simulink model "gm_sampleModel1871_2_sub"  (R2023a)
settings: Solver=VariableStepAuto  StartTime=0.0  StopTime=10.0  RelTol=1e-3
libraries: hdlsllib x1
settings Model: Creator=user1  LastModifiedBy=user1
settings OptimizationCC: BlockReduction=off  ConditionallyExecuteInputs=off
settings DebuggingCC: InheritedTsInSrcMsg=none

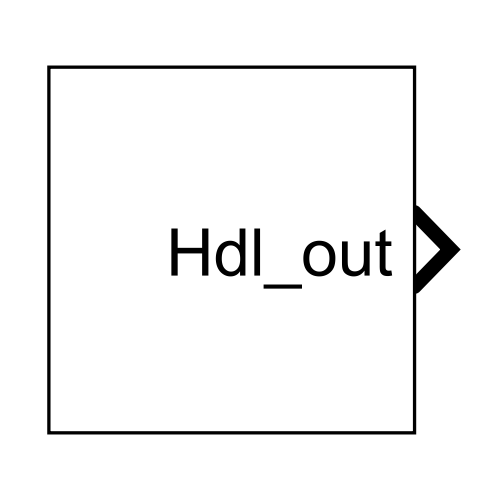
[thumbnail: Simulink's stored preview of the top-level diagram]
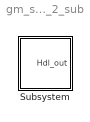
== system gm_sampleModel1871_2_sub ==
  Subsystem : Subsystem

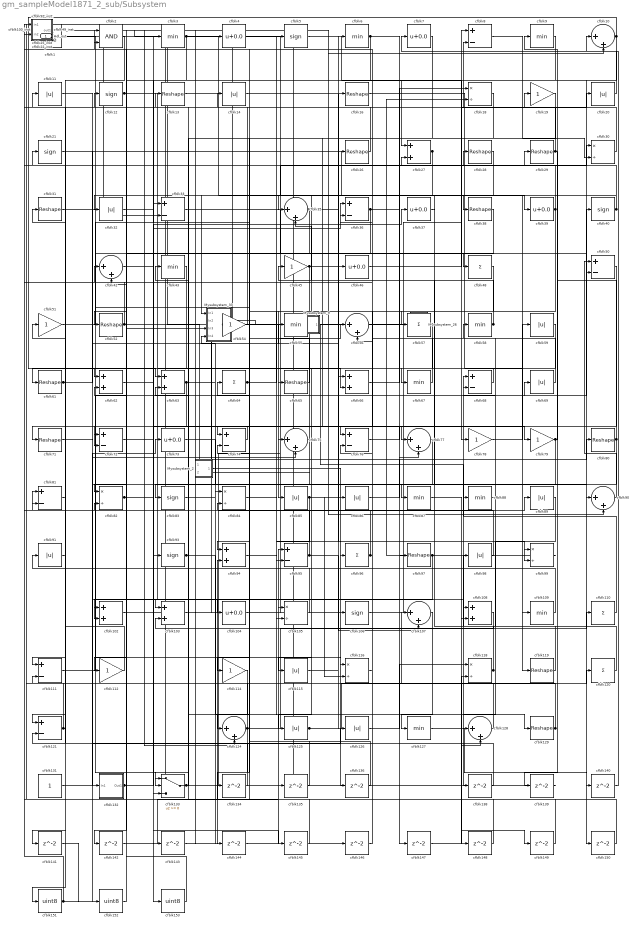
== system gm_sampleModel1871_2_sub/Subsystem ==
  Mysubsystem_2 : Subsystem
  Mysubsystem_26 : Subsystem
  Mysubsystem_33 : Subsystem
  Mysubsystem_9 : Subsystem
  cfblk1 : hdlsllib/Logic and Bit Operations/Bit Slice  lidx=7  ridx=0
  cfblk{10,35,42,56,75,77,90,107,124,128} (10 alike) : Sum  Inputs=|++  OutDataTypeStr=uint8
  cfblk100_inst : Subsystem
  cfblk{27,62..63,66,94,102..103,108} (8 alike) : Sum  OutDataTypeStr=uint8
  cfblk{4,7,37,39,46,73,104} (7 alike) : Bias  Bias=0.0  SaturateOnIntegerOverflow=off
  cfblk{18,30,82,84,99,105,116,118} (8 alike) : Product  Inputs=*/  OutDataTypeStr=uint8  RndMeth=Zero  SaturateOnIntegerOverflow=on
  cfblk{5,12,21,40,83,93,106} (7 alike) : Signum
  cfblk{3,6,9,43,55,58,67,87..88,109,127} (11 alike) : MinMax  OutDataTypeStr=uint8
  cfblk{11,14,20,32,59,69,85..86,89,91,98,115,125..126} (14 alike) : Abs  OutDataTypeStr=uint8  SaturateOnIntegerOverflow=off
  cfblk{48,57,64,96,110,120} (6 alike) : Sum  Inputs=+  OutDataTypeStr=uint8
  cfblk{8,33,36,50,68,72,74,76,81,95,111,121} (12 alike) : Sum  Inputs=+-  OutDataTypeStr=uint8
  cfblk{19,45,51,54,78..79,112,114} (8 alike) : Gain  OutDataTypeStr=uint8
  cfblk{13,16,26,28..29,31,38,52,61,65,71,80,97,119,129} (15 alike) : Reshape
  cfblk122_inst : Subsystem
  cfblk131 : Constant  OutDataTypeStr=uint8  SampleTime=-1
  cfblk132 : Subsystem
  cfblk133 : Switch  OutDataTypeStr=uint8  SaturateOnIntegerOverflow=off  InputSameDT=off
  cfblk{134..136,138..150} (16 alike) : Delay  SampleTime=1
  cfblk151 : DataTypeConversion  OutDataTypeStr=uint8  SaturateOnIntegerOverflow=off  RndMeth=Floor
  cfblk152 : DataTypeConversion  OutDataTypeStr=uint8  SaturateOnIntegerOverflow=off  RndMeth=Floor
  cfblk153 : DataTypeConversion  OutDataTypeStr=uint8  SaturateOnIntegerOverflow=off  RndMeth=Floor
  cfblk2 : Logic  AllPortsSameDT=off  OutDataTypeStr=boolean
  cfblk22_inst : Subsystem
  cfblk25_inst : Subsystem
  cfblk49_inst : Subsystem
  cfblk92_inst : Subsystem
  Hdl_out : Outport  OutDataTypeStr=uint8  SampleTime=1
  wires:
  Mysubsystem_2/1(Out2) -> cfblk136/1
  Mysubsystem_26/1(Out1) -> Mysubsystem_2/2(In2)
  Mysubsystem_33/1(Out1) -> Mysubsystem_2/1(In1)
  Mysubsystem_9/1(Out2) -> cfblk138/1
  cfblk1/1 -> cfblk74/1, cfblk133/2, cfblk116/1
  cfblk10/1 -> cfblk62/1, cfblk27/1, cfblk150/1
  cfblk100_inst/1(out1) -> cfblk90/2, cfblk106/1
  cfblk102/1 -> Mysubsystem_9/1(In2)
  cfblk103/1 -> cfblk56/1
  cfblk104/1 -> cfblk29/1
  cfblk105/1 -> cfblk91/1
  cfblk106/1 -> Mysubsystem_26/1(In1)
  cfblk107/1 -> cfblk127/1
  cfblk108/1 -> cfblk103/2
  cfblk109/1 -> cfblk64/1
  cfblk11/1 -> cfblk132/1(In1)
  cfblk110/1 -> cfblk68/1
  cfblk111/1 -> cfblk40/1
  cfblk112/1 -> cfblk31/1
  cfblk114/1 -> cfblk22_inst/1(in1)
  cfblk115/1 -> cfblk89/1
  cfblk116/1 -> cfblk36/1
  cfblk118/1 -> cfblk98/1, cfblk84/2
  cfblk119/1 -> cfblk45/1
  cfblk12/1 -> cfblk66/2, cfblk148/1
  cfblk120/1 -> cfblk68/2
  cfblk121/1 -> cfblk92_inst/2(in2), cfblk81/1
  cfblk122_inst/1(out1) -> cfblk33/2
  cfblk124/1 -> cfblk51/1, cfblk144/1, cfblk110/1
  cfblk125/1 -> cfblk86/1, cfblk120/1
  cfblk126/1 -> cfblk118/1
  cfblk127/1 -> cfblk140/1
  cfblk128/1 -> cfblk107/1
  cfblk129/1 -> cfblk11/1, Mysubsystem_33/4(In4)
  cfblk13/1 -> cfblk39/1
  cfblk131/1 -> cfblk73/1
  cfblk132/1(Out1) -> cfblk93/1, cfblk37/1
  cfblk133/1 -> cfblk63/2, cfblk16/1
  cfblk134/1 -> cfblk81/2
  cfblk135/1 -> cfblk111/2
  cfblk136/1 -> cfblk22_inst/2(in2)
  cfblk138/1 -> cfblk121/2
  cfblk139/1 -> cfblk1/1
  cfblk14/1 -> cfblk46/1
  cfblk140/1 -> cfblk10/1
  cfblk141/1 -> cfblk152/1
  cfblk142/1 -> cfblk95/1
  cfblk143/1 -> cfblk84/1
  cfblk144/1 -> cfblk105/1
  cfblk145/1 -> cfblk49_inst/1(in1)
  cfblk146/1 -> cfblk76/2
  cfblk147/1 -> cfblk118/2
  cfblk148/1 -> cfblk62/2
  cfblk149/1 -> cfblk94/2
  cfblk150/1 -> cfblk74/2
  cfblk151/1 -> cfblk75/2, cfblk126/1, cfblk100_inst/2(in2)
  cfblk152/1 -> cfblk2/1
  cfblk153/1 -> cfblk2/2
  cfblk16/1 -> cfblk119/1
  cfblk18/1 -> cfblk134/1
  cfblk19/1 -> cfblk103/1
  cfblk2/1 -> cfblk151/1
  cfblk20/1 -> cfblk7/1
  cfblk21/1 -> cfblk77/2
  cfblk22_inst/1(out1) -> cfblk135/1, Mysubsystem_33/3(In3)
  cfblk25_inst/1(out1) -> cfblk124/2
  cfblk26/1 -> cfblk122_inst/2(in2)
  cfblk27/1 -> cfblk85/1, Mysubsystem_33/1(In1)
  cfblk28/1 -> cfblk67/1
  cfblk29/1 -> cfblk8/2, cfblk139/1
  cfblk3/1 -> cfblk38/1, cfblk133/3
  cfblk30/1 -> cfblk14/1
  cfblk31/1 -> cfblk48/1
  cfblk32/1 -> cfblk77/1
  cfblk33/1 -> cfblk97/1
  cfblk35/1 -> cfblk102/2, cfblk30/1
  cfblk36/1 -> cfblk50/2, cfblk142/1
  cfblk37/1 -> cfblk87/1
  cfblk38/1 -> cfblk94/1
  cfblk39/1 -> cfblk95/2, cfblk35/1, cfblk27/2
  cfblk4/1 -> cfblk109/1
  cfblk40/1 -> cfblk49_inst/2(in2), cfblk32/1
  cfblk42/1 -> cfblk143/1
  cfblk43/1 -> cfblk112/1
  cfblk45/1 -> cfblk102/1, cfblk99/2
  cfblk46/1 -> cfblk20/1
  cfblk48/1 -> cfblk76/1
  cfblk49_inst/1(out1) -> cfblk4/1, cfblk25_inst/2(in2), cfblk10/2
  cfblk5/1 -> cfblk78/1
  cfblk50/1 -> cfblk141/1
  cfblk51/1 -> cfblk3/1
  cfblk52/1 -> cfblk92_inst/1(in1), cfblk82/1, cfblk147/1
  cfblk54/1 -> cfblk12/1
  cfblk55/1 -> cfblk100_inst/1(in1), cfblk18/2, Mysubsystem_33/2(In2)
  cfblk56/1 -> cfblk8/1
  cfblk57/1 -> cfblk121/1, Hdl_out/1
  cfblk58/1 -> cfblk35/2, cfblk57/1
  cfblk59/1 -> cfblk125/1
  cfblk6/1 -> cfblk72/2, cfblk108/1
  cfblk61/1 -> cfblk63/1, cfblk26/1, cfblk108/2, cfblk55/1
  cfblk62/1 -> cfblk153/1
  cfblk63/1 -> cfblk72/1, cfblk65/1
  cfblk64/1 -> cfblk5/1, cfblk99/1
  cfblk65/1 -> cfblk33/1
  cfblk66/1 -> cfblk18/1
  cfblk67/1 -> cfblk122_inst/1(in1)
  cfblk68/1 -> cfblk61/1
  cfblk69/1 -> cfblk42/1
  cfblk7/1 -> cfblk75/1
  cfblk71/1 -> cfblk88/1
  cfblk72/1 -> cfblk145/1
  cfblk73/1 -> cfblk90/1
  cfblk74/1 -> cfblk71/1
  cfblk75/1 -> cfblk114/1
  cfblk76/1 -> cfblk79/1
  cfblk77/1 -> cfblk124/1
  cfblk78/1 -> cfblk59/1
  cfblk79/1 -> cfblk133/1, cfblk9/1
  cfblk8/1 -> cfblk30/2
  cfblk80/1 -> cfblk83/1, cfblk19/1
  cfblk81/1 -> cfblk111/1
  cfblk82/1 -> cfblk42/2, cfblk36/2
  cfblk83/1 -> cfblk6/1
  cfblk84/1 -> cfblk96/1
  cfblk85/1 -> cfblk69/1, cfblk116/2, cfblk105/2
  cfblk86/1 -> cfblk80/1
  cfblk87/1 -> cfblk149/1
  cfblk88/1 -> cfblk58/1
  cfblk89/1 -> cfblk128/1
  cfblk9/1 -> cfblk52/1
  cfblk90/1 -> cfblk50/1
  cfblk91/1 -> cfblk21/1
  cfblk92_inst/1(out1) -> cfblk146/1
  cfblk93/1 -> cfblk128/2, cfblk43/1
  cfblk94/1 -> cfblk129/1
  cfblk95/1 -> cfblk28/1, cfblk107/2, cfblk82/2
  cfblk96/1 -> cfblk56/2, cfblk25_inst/1(in1), cfblk13/1
  cfblk97/1 -> cfblk115/1, cfblk104/1
  cfblk98/1 -> cfblk66/1
  cfblk99/1 -> cfblk54/1

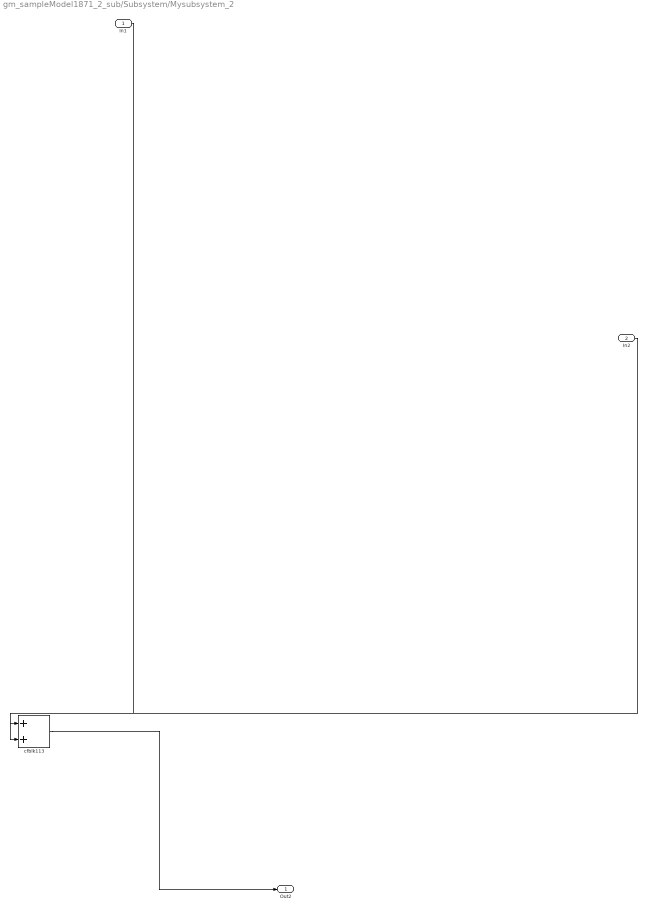
== system gm_sampleModel1871_2_sub/Subsystem/Mysubsystem_2 ==
  In1 : Inport  OutDataTypeStr=uint8  PortDimensions=1  SampleTime=1
  In2 : Inport  Port=2  OutDataTypeStr=uint8  PortDimensions=1  SampleTime=1
  cfblk113 : Sum
  Out2 : Outport  SampleTime=1
  wires:
  In1/1 -> cfblk113/2
  In2/1 -> cfblk113/1
  cfblk113/1 -> Out2/1

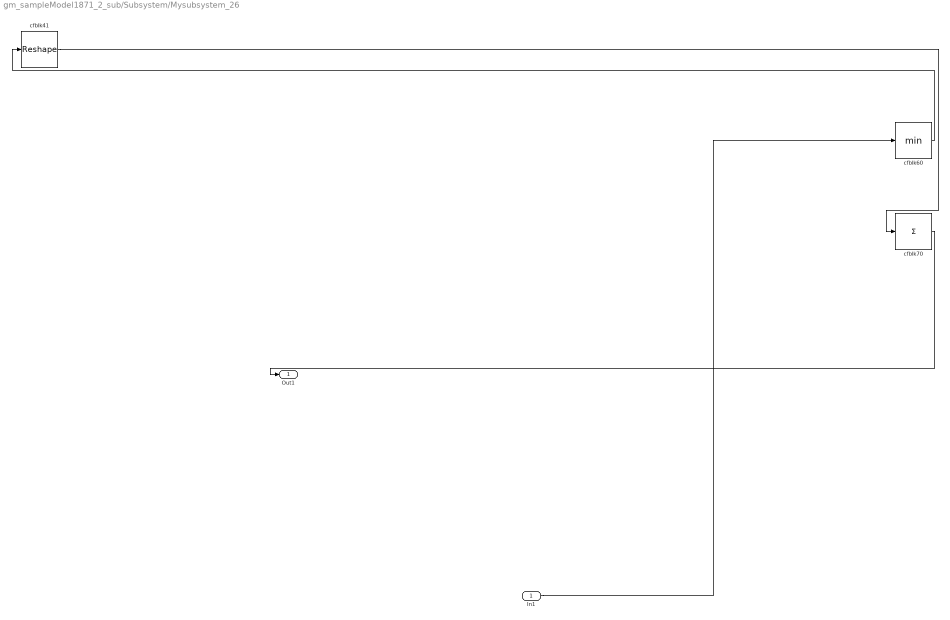
== system gm_sampleModel1871_2_sub/Subsystem/Mysubsystem_26 ==
  In1 : Inport  OutDataTypeStr=uint8  PortDimensions=1  SampleTime=1
  cfblk41 : Reshape
  cfblk60 : MinMax
  cfblk70 : Sum  Inputs=+
  Out1 : Outport  SampleTime=1
  wires:
  In1/1 -> cfblk60/1
  cfblk41/1 -> cfblk70/1
  cfblk60/1 -> cfblk41/1
  cfblk70/1 -> Out1/1

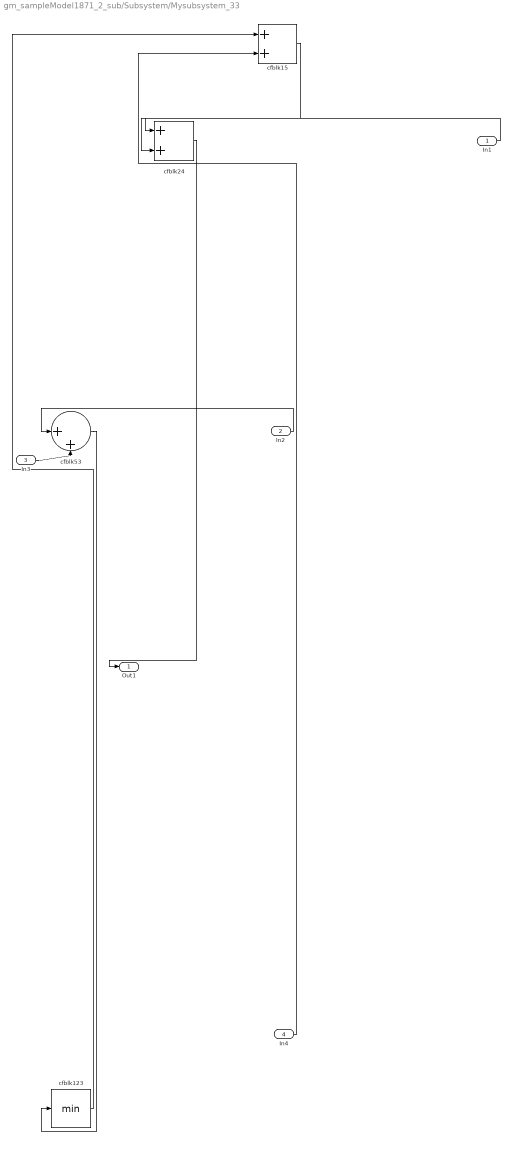
== system gm_sampleModel1871_2_sub/Subsystem/Mysubsystem_33 ==
  In1 : Inport  OutDataTypeStr=uint8  PortDimensions=1  SampleTime=1
  In2 : Inport  Port=2  OutDataTypeStr=uint8  PortDimensions=1  SampleTime=1
  In3 : Inport  Port=3  OutDataTypeStr=uint8  PortDimensions=1  SampleTime=1
  In4 : Inport  Port=4  OutDataTypeStr=uint8  PortDimensions=1  SampleTime=1
  cfblk123 : MinMax
  cfblk15 : Sum
  cfblk24 : Sum
  cfblk53 : Sum  Inputs=|++
  Out1 : Outport  SampleTime=1
  wires:
  In1/1 -> cfblk24/1
  In2/1 -> cfblk53/1
  In3/1 -> cfblk53/2
  In4/1 -> cfblk15/2
  cfblk123/1 -> cfblk15/1
  cfblk15/1 -> cfblk24/2
  cfblk24/1 -> Out1/1
  cfblk53/1 -> cfblk123/1

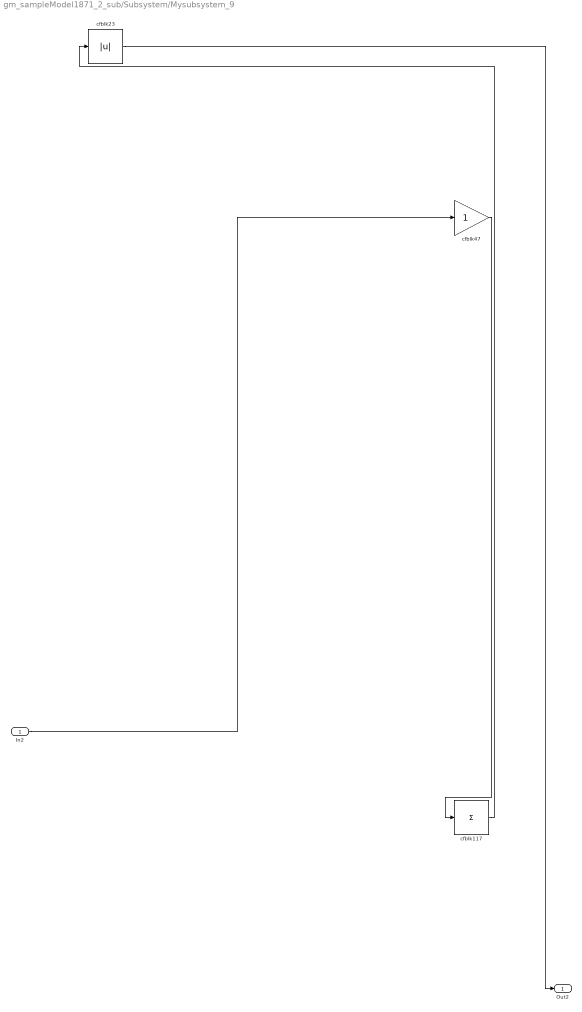
== system gm_sampleModel1871_2_sub/Subsystem/Mysubsystem_9 ==
  In2 : Inport  OutDataTypeStr=uint8  PortDimensions=1  SampleTime=1
  cfblk117 : Sum  Inputs=+
  cfblk23 : Abs  SaturateOnIntegerOverflow=off
  cfblk47 : Gain
  Out2 : Outport  SampleTime=1
  wires:
  In2/1 -> cfblk47/1
  cfblk117/1 -> cfblk23/1
  cfblk23/1 -> Out2/1
  cfblk47/1 -> cfblk117/1

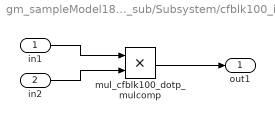
== system gm_sampleModel1871_2_sub/Subsystem/cfblk100_inst ==
  in1 : Inport  OutDataTypeStr=uint8  SampleTime=1
  in2 : Inport  Port=2  OutDataTypeStr=uint8  SampleTime=1
  mul_cfblk100_dotp_mulcomp : Product  Inputs=**  OutDataTypeStr=uint8  SampleTime=1
  out1 : Outport  OutDataTypeStr=uint8  SampleTime=1
  wires:
  in1/1 -> mul_cfblk100_dotp_mulcomp/1
  in2/1 -> mul_cfblk100_dotp_mulcomp/2
  mul_cfblk100_dotp_mulcomp/1 -> out1/1

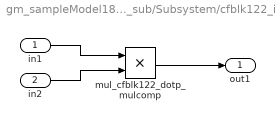
== system gm_sampleModel1871_2_sub/Subsystem/cfblk122_inst ==
  in1 : Inport  OutDataTypeStr=uint8  SampleTime=1
  in2 : Inport  Port=2  OutDataTypeStr=uint8  SampleTime=1
  mul_cfblk122_dotp_mulcomp : Product  Inputs=**  OutDataTypeStr=uint8  SampleTime=1
  out1 : Outport  OutDataTypeStr=uint8  SampleTime=1
  wires:
  in1/1 -> mul_cfblk122_dotp_mulcomp/1
  in2/1 -> mul_cfblk122_dotp_mulcomp/2
  mul_cfblk122_dotp_mulcomp/1 -> out1/1

== system gm_sampleModel1871_2_sub/Subsystem/cfblk132 ==
  In1 : Inport  OutDataTypeStr=uint8  PortDimensions=1  SampleTime=1
  Out1 : Outport  SampleTime=1
  wires:
  In1/1 -> Out1/1

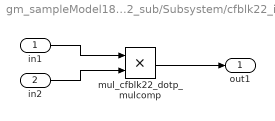
== system gm_sampleModel1871_2_sub/Subsystem/cfblk22_inst ==
  in1 : Inport  OutDataTypeStr=uint8  SampleTime=1
  in2 : Inport  Port=2  OutDataTypeStr=uint8  SampleTime=1
  mul_cfblk22_dotp_mulcomp : Product  Inputs=**  OutDataTypeStr=uint8  SampleTime=1
  out1 : Outport  OutDataTypeStr=uint8  SampleTime=1
  wires:
  in1/1 -> mul_cfblk22_dotp_mulcomp/1
  in2/1 -> mul_cfblk22_dotp_mulcomp/2
  mul_cfblk22_dotp_mulcomp/1 -> out1/1

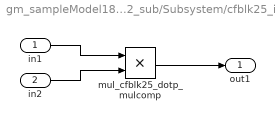
== system gm_sampleModel1871_2_sub/Subsystem/cfblk25_inst ==
  in1 : Inport  OutDataTypeStr=uint8  SampleTime=1
  in2 : Inport  Port=2  OutDataTypeStr=uint8  SampleTime=1
  mul_cfblk25_dotp_mulcomp : Product  Inputs=**  OutDataTypeStr=uint8  SampleTime=1
  out1 : Outport  OutDataTypeStr=uint8  SampleTime=1
  wires:
  in1/1 -> mul_cfblk25_dotp_mulcomp/1
  in2/1 -> mul_cfblk25_dotp_mulcomp/2
  mul_cfblk25_dotp_mulcomp/1 -> out1/1

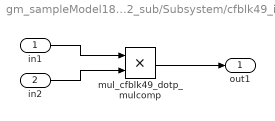
== system gm_sampleModel1871_2_sub/Subsystem/cfblk49_inst ==
  in1 : Inport  OutDataTypeStr=uint8  SampleTime=1
  in2 : Inport  Port=2  OutDataTypeStr=uint8  SampleTime=1
  mul_cfblk49_dotp_mulcomp : Product  Inputs=**  OutDataTypeStr=uint8  SampleTime=1
  out1 : Outport  OutDataTypeStr=uint8  SampleTime=1
  wires:
  in1/1 -> mul_cfblk49_dotp_mulcomp/1
  in2/1 -> mul_cfblk49_dotp_mulcomp/2
  mul_cfblk49_dotp_mulcomp/1 -> out1/1

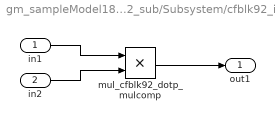
== system gm_sampleModel1871_2_sub/Subsystem/cfblk92_inst ==
  in1 : Inport  OutDataTypeStr=uint8  SampleTime=1
  in2 : Inport  Port=2  OutDataTypeStr=uint8  SampleTime=1
  mul_cfblk92_dotp_mulcomp : Product  Inputs=**  OutDataTypeStr=uint8  SampleTime=1
  out1 : Outport  OutDataTypeStr=uint8  SampleTime=1
  wires:
  in1/1 -> mul_cfblk92_dotp_mulcomp/1
  in2/1 -> mul_cfblk92_dotp_mulcomp/2
  mul_cfblk92_dotp_mulcomp/1 -> out1/1
